simulink model "Forward_Dynamics"  (R2019b)
settings: Solver=VariableStepAuto  StartTime=0.0  StopTime=100  RelTol=1e-3
settings Model: Creator=Stefano  LastModifiedBy=Stefano

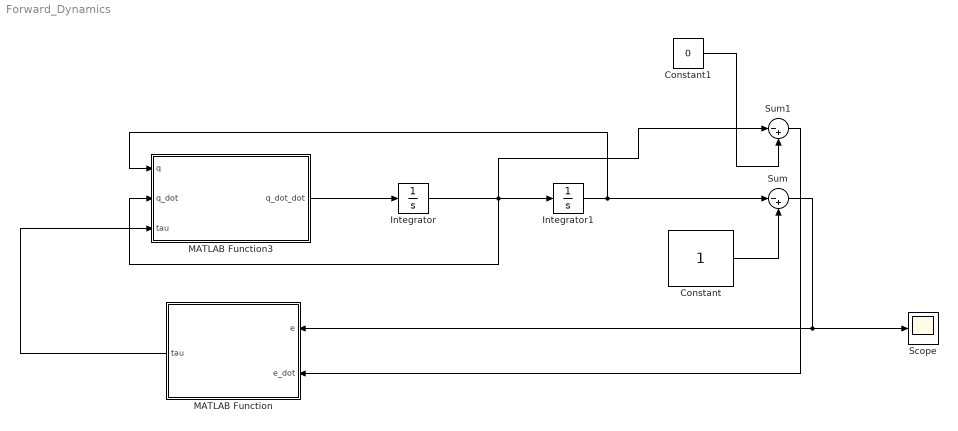
== system Forward_Dynamics ==
  Constant : Constant
  Constant1 : Constant  Value=0
  Integrator : Integrator  InitialCondition=[0,0]'
  Integrator1 : Integrator  InitialCondition=[0,0]'
  MATLAB Function : MATLAB Function  TreatAsAtomicUnit=on
  MATLAB Function3 : MATLAB Function  TreatAsAtomicUnit=on
  Scope : Scope
  Sum : Sum  Inputs=|-+
  Sum1 : Sum  Inputs=|-+
  wires:
  Integrator/1 -> Sum1/1, MATLAB Function3/2(q_dot), Integrator1/1
  MATLAB Function3/1(q_dot_dot) -> Integrator/1
  MATLAB Function/1(tau) -> MATLAB Function3/3(tau)
  Integrator1/1 -> Sum/1, MATLAB Function3/1(q)
  Constant/1 -> Sum/2
  Sum/1 -> Scope/1, MATLAB Function/1(e)
  Constant1/1 -> Sum1/2
  Sum1/1 -> MATLAB Function/2(e_dot)

== matlab function Forward_Dynamics/MATLAB Function ==
  data: e input; tau output; e_dot input
function tau = PD_Controller(e,e_dot)

kd = 2;
kp = 2;
tau = kd*e_dot + kp*e;
end

== matlab function Forward_Dynamics/MATLAB Function3 ==
  data: q input; q_dot_dot output; q_dot input; tau input
function q_dot_dot = fcn(q,q_dot,tau)

m1 = 1;
m2 = 1;

l1=1;
l2=1;

r1=l1/2;
r2=l2/2;


Izz1 = (1/12)*m1*l1^2;
Izz2 = (1/12)*m2*l2^2;



Alpha = Izz1 + Izz2 + m1*(r1)^2 + m2*(l1^2+r2^2);
Beta = m2*l1*r2;
Delta = Izz2 +m2*r2^2;

M = [Alpha + 2* Beta *cos(q(2)), Delta + Beta *cos(q(2));
     Delta + Beta *cos(q(2)),    Delta];

C = [-Beta*sin(q(2))*q_dot(2), -Beta*sin(q(2))*(q_dot(1)+q_dot(2));
     Beta*sin(q(2))*q_dot(1),   0];



q_dot_dot = inv(M)*([tau(1); tau(2)]- C*[q_dot(1); q_dot(2)]);
